simulink library "asbhl20screen"  (R2016b)
settings: Solver=ode45  StartTime=0.0  StopTime=10.0  RelTol=1e-3
undefined symbols (not defined in the file): Tf, Tfg
Description:
  | HL-20 control surface and hydraulic system monitoring modules
settings Model: ExtModeAutoUpdateStatusClock=off  Creator=The MathWorks, Inc.  LastModifiedBy=The MathWorks, Inc.
settings DataIOCC: LimitDataPoints=on  SaveFormat=Array  SignalLoggingSaveFormat=ModelDataLogs
settings OptimizationCC: BlockReduction=off  BooleanDataType=off  ExpressionDepthLimit=2147483647  LifeSpan=inf
settings DebuggingCC: SaveWithParameterizedLinksMsg=none  UnderspecifiedInitializationDetection=Classic  MergeDetectMultiDrivingBlocksExec=none  SignalResolutionControl=TryResolveAllWithWarning  FcnCallInpInsideContextMsg=warning  StateNameClashWarn=warning  StrictBusMsg=Warning  SFUnexpectedBacktrackingDiag=warning  SFNoUnconditionalDefaultTransitionDiag=warning  SFExecutionAtInitializationDiag=none
settings HardwareCC: ProdBitPerPointer=32  ProdBitPerSizeT=32  ProdBitPerPtrDiffT=32  ProdLargestAtomicFloat=None  ProdIntDivRoundTo=Undefined  ProdEndianess=Unspecified  ProdWordSize=32  ProdHWDeviceType=32-bit Generic  TargetUnknown=on
settings ModelReferenceCC: PropagateSignalLabelsOutOfModel=off
settings GRTTargetCC: TargetLangStandard=C89/C90 (ANSI)  GeneratePreprocessorConditionals=Disable all  CombineOutputUpdateFcns=off  GRTInterface=on
settings ConfigComp: CovMetricSettings=dw  CovHtmlReporting=on  CovSaveCumulativeToWorkspaceVar=on  CovSaveSingleToWorkspaceVar=on  CovExternalEMLEnable=off  CovSFcnEnable=off

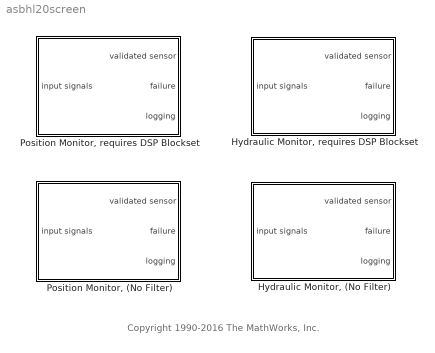
== system asbhl20screen ==
  note: Copyright 1990-2016 The MathWorks, Inc.
  "Hydraulic Monitor, (No Filter)" : Subsystem
  "Hydraulic Monitor, requires DSP Blockset" : Subsystem
  "Position Monitor, (No Filter)" : Subsystem
  "Position Monitor, requires DSP Blockset" : Subsystem

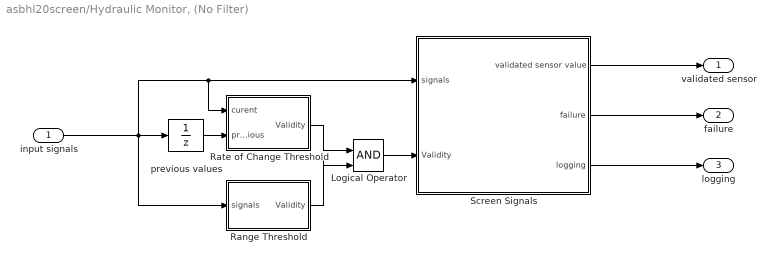
== system asbhl20screen/Hydraulic Monitor, (No Filter) ==
  input signals : Inport  PortDimensions=3  SampleTime=Tf
  Logical Operator : Logic  IconShape=distinctive  AllPortsSameDT=off
  Range Threshold : Subsystem
  Rate of Change Threshold : Subsystem
  Screen Signals : Subsystem
  previous values : UnitDelay  SampleTime=-1
  validated sensor : Outport
  failure : Outport  Port=2
  logging : Outport  Port=3
  wires:
  Screen Signals/3(logging) -> logging/1
  Logical Operator/1 -> Screen Signals/2(Validity)
  Rate of Change Threshold/1(Validity) -> Logical Operator/1
  Range Threshold/1(Validity) -> Logical Operator/2
  previous values/1 -> Rate of Change Threshold/2(previous)
  Screen Signals/1(validated sensor value) -> validated sensor/1
  input signals/1 -> Range Threshold/1(signals), Screen Signals/1(signals), Rate of Change Threshold/1(curent), previous values/1
  Screen Signals/2(failure) -> failure/1

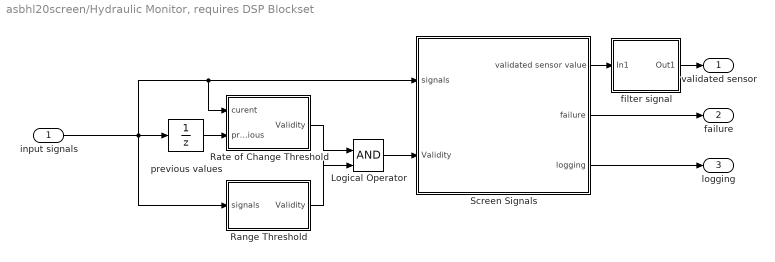
== system asbhl20screen/Hydraulic Monitor, requires DSP Blockset ==
  input signals : Inport  PortDimensions=3  SampleTime=Tf
  Logical Operator : Logic  IconShape=distinctive  AllPortsSameDT=off
  Range Threshold : Subsystem
  Rate of Change Threshold : Subsystem
  Screen Signals : Subsystem
  filter signal : Subsystem
  previous values : UnitDelay  SampleTime=-1
  validated sensor : Outport
  failure : Outport  Port=2
  logging : Outport  Port=3
  wires:
  Screen Signals/2(failure) -> failure/1
  input signals/1 -> previous values/1, Rate of Change Threshold/1(curent), Screen Signals/1(signals), Range Threshold/1(signals)
  Screen Signals/1(validated sensor value) -> filter signal/1(In1)
  previous values/1 -> Rate of Change Threshold/2(previous)
  Range Threshold/1(Validity) -> Logical Operator/2
  Rate of Change Threshold/1(Validity) -> Logical Operator/1
  Logical Operator/1 -> Screen Signals/2(Validity)
  filter signal/1(Out1) -> validated sensor/1
  Screen Signals/3(logging) -> logging/1

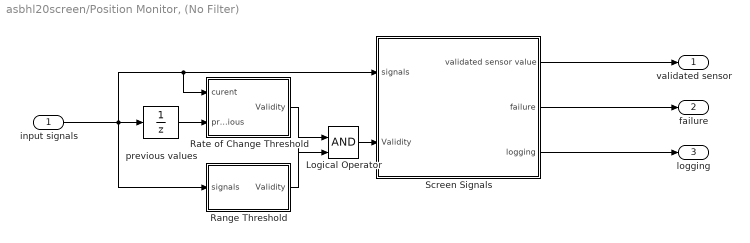
== system asbhl20screen/Position Monitor, (No Filter) ==
  input signals : Inport  PortDimensions=3  SampleTime=Tf
  Logical Operator : Logic  IconShape=distinctive  AllPortsSameDT=off
  Range Threshold : Subsystem
  Rate of Change Threshold : Subsystem
  Screen Signals : Subsystem
  previous values : UnitDelay  SampleTime=-1
  validated sensor : Outport
  failure : Outport  Port=2
  logging : Outport  Port=3
  wires:
  Screen Signals/3(logging) -> logging/1
  Screen Signals/2(failure) -> failure/1
  input signals/1 -> Range Threshold/1(signals), previous values/1, Screen Signals/1(signals), Rate of Change Threshold/1(curent)
  Screen Signals/1(validated sensor value) -> validated sensor/1
  previous values/1 -> Rate of Change Threshold/2(previous)
  Range Threshold/1(Validity) -> Logical Operator/2
  Rate of Change Threshold/1(Validity) -> Logical Operator/1
  Logical Operator/1 -> Screen Signals/2(Validity)

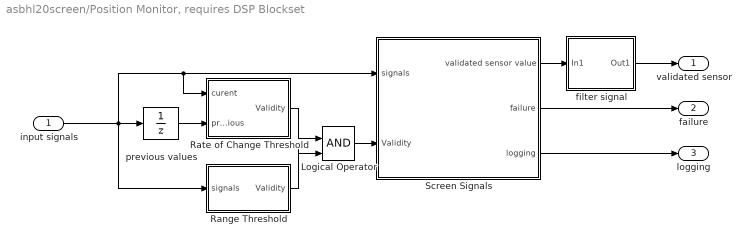
== system asbhl20screen/Position Monitor, requires DSP Blockset ==
  input signals : Inport  PortDimensions=3  SampleTime=Tf
  Logical Operator : Logic  IconShape=distinctive  AllPortsSameDT=off
  Range Threshold : Subsystem
  Rate of Change Threshold : Subsystem
  Screen Signals : Subsystem
  filter signal : Subsystem
  previous values : UnitDelay  SampleTime=-1
  validated sensor : Outport
  failure : Outport  Port=2
  logging : Outport  Port=3
  wires:
  Logical Operator/1 -> Screen Signals/2(Validity)
  Rate of Change Threshold/1(Validity) -> Logical Operator/1
  Range Threshold/1(Validity) -> Logical Operator/2
  previous values/1 -> Rate of Change Threshold/2(previous)
  Screen Signals/1(validated sensor value) -> filter signal/1(In1)
  input signals/1 -> Rate of Change Threshold/1(curent), Screen Signals/1(signals), previous values/1, Range Threshold/1(signals)
  Screen Signals/2(failure) -> failure/1
  Screen Signals/3(logging) -> logging/1
  filter signal/1(Out1) -> validated sensor/1

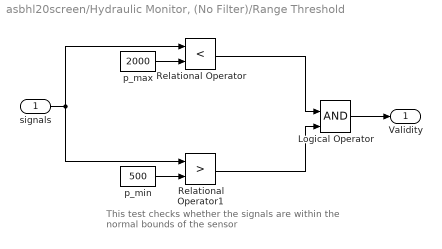
== system asbhl20screen/Hydraulic Monitor, (No Filter)/Range Threshold ==
  note: This test checks whether the signals are within
      | the normal bounds of the sensor
  signals : Inport
  Logical Operator : Logic  IconShape=distinctive  AllPortsSameDT=off
  Relational Operator : RelationalOperator  Operator=<  RndMeth=Nearest
  Relational Operator1 : RelationalOperator  Operator=>  RndMeth=Nearest
  p_max : Constant  Value=2000
  p_min : Constant  Value=500
  Validity : Outport
  wires:
  Logical Operator/1 -> Validity/1
  p_min/1 -> Relational Operator1/2
  p_max/1 -> Relational Operator/2
  Relational Operator1/1 -> Logical Operator/2
  Relational Operator/1 -> Logical Operator/1
  signals/1 -> Relational Operator1/1, Relational Operator/1

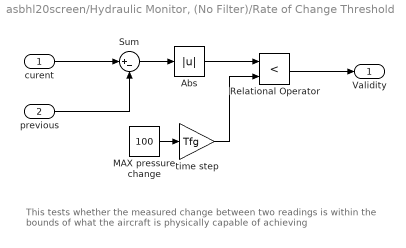
== system asbhl20screen/Hydraulic Monitor, (No Filter)/Rate of Change Threshold ==
  note: This tests whether the measured change between two readings
      | is within the bounds of what the aircraft is physically capable of achieving
  curent : Inport
  previous : Inport  Port=2
  Abs : Abs  SaturateOnIntegerOverflow=on
  MAX pressure change : Constant  Value=100
  Relational Operator : RelationalOperator  Operator=<  OutDataTypeStr=boolean  RndMeth=Nearest
  Sum : Sum  Inputs=|+-  SaturateOnIntegerOverflow=on
  time step : Gain  Gain=Tfg  SaturateOnIntegerOverflow=on  OutDataTypeStr=Inherit: Same as input  ParamDataTypeStr=Inherit: Same as input
  Validity : Outport
  wires:
  Sum/1 -> Abs/1
  time step/1 -> Relational Operator/2
  MAX pressure change/1 -> time step/1
  Relational Operator/1 -> Validity/1
  previous/1 -> Sum/2
  curent/1 -> Sum/1
  Abs/1 -> Relational Operator/1

== system asbhl20screen/Hydraulic Monitor, (No Filter)/Screen Signals ==
  signals : Inport
  Validity : Inport  Port=2
  screen logic : Stateflow chart  TreatAsAtomicUnit=on
  validated sensor value : Outport
  failure : Outport  Port=2
  logging : Outport  Port=3
  wires:
  screen logic/3(" logging") -> logging/1
  signals/1 -> screen logic/1(signals)
  Validity/1 -> screen logic/2(validity)
  screen logic/1(valid_signal) -> validated sensor value/1
  screen logic/2(failure) -> failure/1

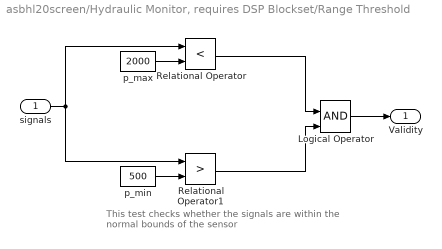
== system asbhl20screen/Hydraulic Monitor, requires DSP Blockset/Range Threshold ==
  note: This test checks whether the signals are within
      | the normal bounds of the sensor
  signals : Inport
  Logical Operator : Logic  IconShape=distinctive  AllPortsSameDT=off
  Relational Operator : RelationalOperator  Operator=<  RndMeth=Nearest
  Relational Operator1 : RelationalOperator  Operator=>  RndMeth=Nearest
  p_max : Constant  Value=2000
  p_min : Constant  Value=500
  Validity : Outport
  wires:
  signals/1 -> Relational Operator/1, Relational Operator1/1
  Relational Operator/1 -> Logical Operator/1
  Relational Operator1/1 -> Logical Operator/2
  p_max/1 -> Relational Operator/2
  p_min/1 -> Relational Operator1/2
  Logical Operator/1 -> Validity/1

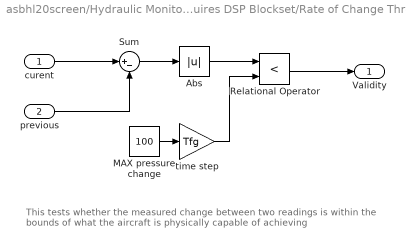
== system asbhl20screen/Hydraulic Monitor, requires DSP Blockset/Rate of Change Threshold ==
  note: This tests whether the measured change between two readings
      | is within the bounds of what the aircraft is physically capable of achieving
  curent : Inport
  previous : Inport  Port=2
  Abs : Abs  SaturateOnIntegerOverflow=on
  MAX pressure change : Constant  Value=100
  Relational Operator : RelationalOperator  Operator=<  OutDataTypeStr=boolean  RndMeth=Nearest
  Sum : Sum  Inputs=|+-  SaturateOnIntegerOverflow=on
  time step : Gain  Gain=Tfg  SaturateOnIntegerOverflow=on  OutDataTypeStr=Inherit: Same as input  ParamDataTypeStr=Inherit: Same as input
  Validity : Outport
  wires:
  curent/1 -> Sum/1
  previous/1 -> Sum/2
  Relational Operator/1 -> Validity/1
  MAX pressure change/1 -> time step/1
  time step/1 -> Relational Operator/2
  Sum/1 -> Abs/1
  Abs/1 -> Relational Operator/1

== system asbhl20screen/Hydraulic Monitor, requires DSP Blockset/Screen Signals ==
  signals : Inport
  Validity : Inport  Port=2
  screen logic : Stateflow chart  TreatAsAtomicUnit=on
  validated sensor value : Outport
  failure : Outport  Port=2
  logging : Outport  Port=3
  wires:
  screen logic/2(failure) -> failure/1
  screen logic/1(valid_signal) -> validated sensor value/1
  Validity/1 -> screen logic/2(validity)
  signals/1 -> screen logic/1(signals)
  screen logic/3(" logging") -> logging/1

== system asbhl20screen/Hydraulic Monitor, requires DSP Blockset/filter signal ==
  In1 : Inport
  Discrete FIR Filter : DiscreteFir  Coefficients=[0.1832 0.3168 0.3168 0.1832]  AccumDataTypeStr=Inherit: Same as product output  OutDataTypeStr=Inherit: Same as input
  Out1 : Outport
  wires:
  In1/1 -> Discrete FIR Filter/1
  Discrete FIR Filter/1 -> Out1/1

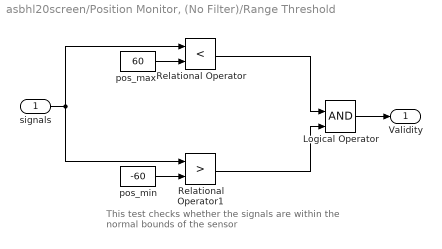
== system asbhl20screen/Position Monitor, (No Filter)/Range Threshold ==
  note: This test checks whether the signals are within
      | the normal bounds of the sensor
  signals : Inport
  Logical Operator : Logic  IconShape=distinctive  AllPortsSameDT=off
  Relational Operator : RelationalOperator  Operator=<  RndMeth=Nearest
  Relational Operator1 : RelationalOperator  Operator=>  RndMeth=Nearest
  pos_max : Constant  Value=60
  pos_min : Constant  Value=-60
  Validity : Outport
  wires:
  Logical Operator/1 -> Validity/1
  pos_min/1 -> Relational Operator1/2
  pos_max/1 -> Relational Operator/2
  Relational Operator1/1 -> Logical Operator/2
  Relational Operator/1 -> Logical Operator/1
  signals/1 -> Relational Operator1/1, Relational Operator/1

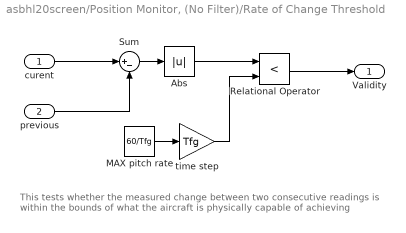
== system asbhl20screen/Position Monitor, (No Filter)/Rate of Change Threshold ==
  note: This tests whether the measured change between two consecutive readings
      | is within the bounds of what the aircraft is physically capable of achieving
  curent : Inport
  previous : Inport  Port=2
  Abs : Abs  SaturateOnIntegerOverflow=on
  MAX pitch rate : Constant  Value=60/Tfg
  Relational Operator : RelationalOperator  Operator=<  OutDataTypeStr=boolean  RndMeth=Nearest
  Sum : Sum  Inputs=|+-  SaturateOnIntegerOverflow=on
  time step : Gain  Gain=Tfg  SaturateOnIntegerOverflow=on  OutDataTypeStr=Inherit: Same as input  ParamDataTypeStr=Inherit: Same as input
  Validity : Outport
  wires:
  curent/1 -> Sum/1
  previous/1 -> Sum/2
  Relational Operator/1 -> Validity/1
  MAX pitch rate/1 -> time step/1
  time step/1 -> Relational Operator/2
  Sum/1 -> Abs/1
  Abs/1 -> Relational Operator/1

== system asbhl20screen/Position Monitor, (No Filter)/Screen Signals ==
  signals : Inport
  Validity : Inport  Port=2
  screen logic : Stateflow chart  TreatAsAtomicUnit=on
  validated sensor value : Outport
  failure : Outport  Port=2
  logging : Outport  Port=3
  wires:
  screen logic/3(" logging") -> logging/1
  screen logic/2(failure) -> failure/1
  screen logic/1(valid_signal) -> validated sensor value/1
  Validity/1 -> screen logic/2(validity)
  signals/1 -> screen logic/1(signals)

== system asbhl20screen/Position Monitor, requires DSP Blockset/Range Threshold ==
  note: This test checks whether the signals are within
      | the normal bounds of the sensor
  signals : Inport
  Logical Operator : Logic  IconShape=distinctive  AllPortsSameDT=off
  Relational Operator : RelationalOperator  Operator=<  RndMeth=Nearest
  Relational Operator1 : RelationalOperator  Operator=>  RndMeth=Nearest
  pos_max : Constant  Value=60
  pos_min : Constant  Value=-60
  Validity : Outport
  wires:
  signals/1 -> Relational Operator/1, Relational Operator1/1
  Relational Operator/1 -> Logical Operator/1
  Relational Operator1/1 -> Logical Operator/2
  pos_max/1 -> Relational Operator/2
  pos_min/1 -> Relational Operator1/2
  Logical Operator/1 -> Validity/1

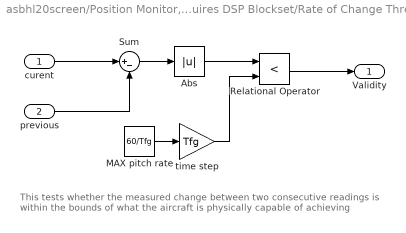
== system asbhl20screen/Position Monitor, requires DSP Blockset/Rate of Change Threshold ==
  note: This tests whether the measured change between two consecutive readings
      | is within the bounds of what the aircraft is physically capable of achieving
  curent : Inport
  previous : Inport  Port=2
  Abs : Abs  SaturateOnIntegerOverflow=on
  MAX pitch rate : Constant  Value=60/Tfg
  Relational Operator : RelationalOperator  Operator=<  OutDataTypeStr=boolean  RndMeth=Nearest
  Sum : Sum  Inputs=|+-  SaturateOnIntegerOverflow=on
  time step : Gain  Gain=Tfg  SaturateOnIntegerOverflow=on  OutDataTypeStr=Inherit: Same as input  ParamDataTypeStr=Inherit: Same as input
  Validity : Outport
  wires:
  Sum/1 -> Abs/1
  time step/1 -> Relational Operator/2
  MAX pitch rate/1 -> time step/1
  Relational Operator/1 -> Validity/1
  previous/1 -> Sum/2
  curent/1 -> Sum/1
  Abs/1 -> Relational Operator/1

== system asbhl20screen/Position Monitor, requires DSP Blockset/Screen Signals ==
  signals : Inport
  Validity : Inport  Port=2
  screen logic : Stateflow chart  TreatAsAtomicUnit=on
  validated sensor value : Outport
  failure : Outport  Port=2
  logging : Outport  Port=3
  wires:
  signals/1 -> screen logic/1(signals)
  Validity/1 -> screen logic/2(validity)
  screen logic/1(valid_signal) -> validated sensor value/1
  screen logic/2(failure) -> failure/1
  screen logic/3(" logging") -> logging/1

== system asbhl20screen/Position Monitor, requires DSP Blockset/filter signal ==
  In1 : Inport
  Discrete FIR Filter : DiscreteFir  Coefficients=[0.1832 0.3168 0.3168 0.1832]  AccumDataTypeStr=Inherit: Same as product output  OutDataTypeStr=Inherit: Same as input
  Out1 : Outport
  wires:
  In1/1 -> Discrete FIR Filter/1
  Discrete FIR Filter/1 -> Out1/1

== stateflow chart asbhl20screen/Position Monitor, (No Filter)/Screen Signals/screen logic ==
  state Screen [parallel]
    settings: executionOrder=1
    note: no valid signals
    state three
      (default) -> (junction 86) : {sum=signals[1]+signals[2]+signals[3];}
      (junction 86) -> (junction 103) : {middle=sum-...
          | max(max(signals[1],signals[2]),signals[3])-...
          | min(min(signals[1],signals[2]),signals[3]);}
      (junction 103) -> (junction 109) [order 1] : [bad==1]
      (junction 109) -> (junction 100) : {none();}
      (junction 103) -> (junction 85) [order 2] : {valid_signal=middle;}
      (junction 85) -> (junction 87) : {failure=0;}
      (junction 87) -> (junction 88) : {prev_signal=valid_signal;}
      (junction 88) -> (junction 108) : {count=0;}
    state zero
      (default) -> (junction 99) : {none();}
    state one
      note: Only one valid sensor - just use the valid signal.
          | Failure is false
      (default) -> (junction 111) : {valid_signal=signals[select[1]];}
      (junction 111) -> (junction 112) : {failure=0;}
      (junction 112) -> (junction 113) : {prev_signal=valid_signal;}
      (junction 113) -> (junction 110) : {count=0;}
    state two
      (default) -> (junction 102) : {diff=abs(signals[select[1]]-signals[select[2]]);}
      (junction 102) -> (junction 107) [order 1] : [diff>diff_max]
      (junction 102) -> (junction 98) [order 2] : {mean=(signals[select[1]]+signals[select[2]])/2;}
      (junction 107) -> (junction 101) : {none();}
      (junction 98) -> (junction 97) : {valid_signal=mean;}
      (junction 97) -> (junction 95) : {failure=0;}
      (junction 95) -> (junction 94) : {prev_signal=valid_signal;}
      (junction 94) -> (junction 106) : {count=0;}
    (default) -> (junction 84) : {n=valid_sensors();}
    three -> Screen
    (junction 84) -> zero [order 4]
    (junction 84) -> three [order 1] : [n==3]
    zero -> Screen
    (junction 84) -> two [order 2] : [n==2]
    (junction 84) -> one [order 3] : [n==1]
    one -> Screen
    two -> Screen
  state failure_logging [parallel]
    settings: executionOrder=2
    state off
    state logging
    off -> logging : log
    logging -> logging [order 2] : log
    (default) -> off
    logging -> off [order 1] : after(30,tick)[~failure]
  state num = valid_sensors() [function]
    (default) -> (junction 228)
    (junction 228) -> (junction 230) : { aVarTruthTableCondition_1 = (validity[1] == 1); }
    (junction 230) -> (junction 232) : { aVarTruthTableCondition_2 = (validity[2] == 1); }
    (junction 232) -> (junction 234) : { aVarTruthTableCondition_3 = (validity[3] == 1); }
    (junction 234) -> (junction 236) [order 1] : [aVarTruthTableCondition_1 && aVarTruthTableCondition_2 && aVarTruthTableCondition_3]
    (junction 236) -> (junction 238) : {
        | /* All 3 signals valid */
        | num = 3;
        | }
    (junction 234) -> (junction 240) [order 2]
    (junction 240) -> (junction 242) [order 1] : [aVarTruthTableCondition_1 && aVarTruthTableCondition_2 && !aVarTruthTableCondition_3]
    (junction 242) -> (junction 244) : {
        | /* Signals 1&2 valid */
        | num = 2;
        | select[1]=1;
        | select[2]=2;
        | }
    (junction 240) -> (junction 246) [order 2]
    (junction 246) -> (junction 248) [order 1] : [aVarTruthTableCondition_1 && !aVarTruthTableCondition_2 && aVarTruthTableCondition_3]
    (junction 248) -> (junction 250) : {
        | /* Signals 1&3 valid */
        | num = 2;
        | select[1]=1;
        | select[2]=3;
        | }
    (junction 246) -> (junction 252) [order 2]
    (junction 252) -> (junction 254) [order 1] : [aVarTruthTableCondition_1 && !aVarTruthTableCondition_2 && !aVarTruthTableCondition_3]
    (junction 254) -> (junction 256) : {
        | /* Signal 1 valid */
        | num = 1;
        | select[1]=1;
        | select[2]=0;
        | }
    (junction 252) -> (junction 258) [order 2]
    (junction 258) -> (junction 260) [order 1] : [!aVarTruthTableCondition_1 && aVarTruthTableCondition_2 && aVarTruthTableCondition_3]
    (junction 260) -> (junction 262) : {
        | /* Signals 2&3 valid */
        | num = 2;
        | select[1]=2;
        | select[2]=3;
        | }
    (junction 258) -> (junction 264) [order 2]
    (junction 264) -> (junction 266) [order 1] : [!aVarTruthTableCondition_1 && aVarTruthTableCondition_2 && !aVarTruthTableCondition_3]
    (junction 266) -> (junction 268) : {
        | /* Signal 2 valid */
        | num = 1;
        | select[1]=2;
        | select[2]=0;
        | }
    (junction 264) -> (junction 270) [order 2]
    (junction 270) -> (junction 272) [order 1] : [!aVarTruthTableCondition_1 && !aVarTruthTableCondition_2 && aVarTruthTableCondition_3]
    (junction 272) -> (junction 274) : {
        | /* Signal 3 valid */
        | num = 1;
        | select[1]=3;
        | select[2]=0;
        | }
    (junction 270) -> (junction 276) [order 2]
    (junction 276) -> (junction 278) [order 1] : [!aVarTruthTableCondition_1 && !aVarTruthTableCondition_2 && !aVarTruthTableCondition_3]
    (junction 278) -> (junction 280) : {
        | /* 'None':no signals valid */
        | num = 0;
        | }
    (junction 276) -> (junction 282) [order 2]
  state none() [function]
    (default) -> (junction 93)
    (junction 93) -> (junction 91) : {count=count+1;}
    (junction 91) -> (junction 104) [order 1] : [count>3]
    (junction 104) -> (junction 92) : {count=3;}
    (junction 92) -> (junction 89) : {valid_signal=0;}
    (junction 91) -> (junction 90) [order 2] : {valid_signal=prev_signal;}
    (junction 89) -> (junction 105) : {failure=1;}
    (junction 90) -> (junction 96) : {failure=0;}
    (junction 96) -> (junction 105) : {send(log,failure_logging)}
  data: middle local double; sum local double; diff local double; mean local double; num function_output int8; aVarTruthTableCondition_1 temporary boolean =0; aVarTruthTableCondition_2 temporary boolean =0; aVarTruthTableCondition_3 temporary boolean =0; signals input double size=3; validity input boolean size=3; n local int8; valid_signal output double; failure output boolean; prev_signal local double; count local int8; diff_max constant double =3; bad local boolean; select local int8 size=2; logging output unknown
  events: log local EITHER_EDGE_EVENT

== stateflow chart asbhl20screen/Hydraulic Monitor, (No Filter)/Screen Signals/screen logic ==
  state Screen [parallel]
    settings: executionOrder=1
    note: no valid signals
    state three
      (default) -> (junction 94) : {sum=signals[1]+signals[2]+signals[3];}
      (junction 94) -> (junction 97) : {middle=sum-...
          | max(max(signals[1],signals[2]),signals[3])-...
          | min(min(signals[1],signals[2]),signals[3]);}
      (junction 97) -> (junction 95) [order 1] : [bad==1]
      (junction 95) -> (junction 98) : {none();}
      (junction 97) -> (junction 101) [order 2] : {valid_signal=middle;}
      (junction 101) -> (junction 102) : {failure=0;}
      (junction 102) -> (junction 107) : {prev_signal=valid_signal;}
      (junction 107) -> (junction 110) : {count=0;}
    state zero
      (default) -> (junction 113) : {none();}
    state one
      note: Only one valid sensor - just use the valid signal.
          | Failure is false
      (default) -> (junction 112) : {valid_signal=signals[select[1]];}
      (junction 112) -> (junction 111) : {failure=0;}
      (junction 111) -> (junction 99) : {prev_signal=valid_signal;}
      (junction 99) -> (junction 108) : {count=0;}
    state two
      (default) -> (junction 87) : {diff=abs(signals[select[1]]-signals[select[2]]);}
      (junction 87) -> (junction 88) [order 1] : [diff>diff_max]
      (junction 87) -> (junction 100) [order 2] : {mean=(signals[select[1]]+signals[select[2]])/2;}
      (junction 88) -> (junction 85) : {none();}
      (junction 100) -> (junction 103) : {valid_signal=mean;}
      (junction 103) -> (junction 109) : {failure=0;}
      (junction 109) -> (junction 86) : {prev_signal=valid_signal;}
      (junction 86) -> (junction 84) : {count=0;}
    (default) -> (junction 106) : {n=valid_sensors();}
    three -> Screen
    (junction 106) -> zero [order 4]
    (junction 106) -> three [order 1] : [n==3]
    zero -> Screen
    (junction 106) -> two [order 2] : [n==2]
    (junction 106) -> one [order 3] : [n==1]
    one -> Screen
    two -> Screen
  state failure_logging [parallel]
    settings: executionOrder=2
    state off
    state logging
    off -> logging : log
    logging -> logging [order 2] : log
    (default) -> off
    logging -> off [order 1] : after(30,tick)[~failure]
  state num = valid_sensors() [function]
    (default) -> (junction 228)
    (junction 228) -> (junction 230) : { aVarTruthTableCondition_1 = (validity[1] == 1); }
    (junction 230) -> (junction 232) : { aVarTruthTableCondition_2 = (validity[2] == 1); }
    (junction 232) -> (junction 234) : { aVarTruthTableCondition_3 = (validity[3] == 1); }
    (junction 234) -> (junction 236) [order 1] : [aVarTruthTableCondition_1 && aVarTruthTableCondition_2 && aVarTruthTableCondition_3]
    (junction 236) -> (junction 238) : {
        | /* All 3 signals valid */
        | num = 3;
        | }
    (junction 234) -> (junction 240) [order 2]
    (junction 240) -> (junction 242) [order 1] : [aVarTruthTableCondition_1 && aVarTruthTableCondition_2 && !aVarTruthTableCondition_3]
    (junction 242) -> (junction 244) : {
        | /* Signals 1&2 valid */
        | num = 2;
        | select[1]=1;
        | select[2]=2;
        | }
    (junction 240) -> (junction 246) [order 2]
    (junction 246) -> (junction 248) [order 1] : [aVarTruthTableCondition_1 && !aVarTruthTableCondition_2 && aVarTruthTableCondition_3]
    (junction 248) -> (junction 250) : {
        | /* Signals 1&3 valid */
        | num = 2;
        | select[1]=1;
        | select[2]=3;
        | }
    (junction 246) -> (junction 252) [order 2]
    (junction 252) -> (junction 254) [order 1] : [aVarTruthTableCondition_1 && !aVarTruthTableCondition_2 && !aVarTruthTableCondition_3]
    (junction 254) -> (junction 256) : {
        | /* Signal 1 valid */
        | num = 1;
        | select[1]=1;
        | select[2]=0;
        | }
    (junction 252) -> (junction 258) [order 2]
    (junction 258) -> (junction 260) [order 1] : [!aVarTruthTableCondition_1 && aVarTruthTableCondition_2 && aVarTruthTableCondition_3]
    (junction 260) -> (junction 262) : {
        | /* Signals 2&3 valid */
        | num = 2;
        | select[1]=2;
        | select[2]=3;
        | }
    (junction 258) -> (junction 264) [order 2]
    (junction 264) -> (junction 266) [order 1] : [!aVarTruthTableCondition_1 && aVarTruthTableCondition_2 && !aVarTruthTableCondition_3]
    (junction 266) -> (junction 268) : {
        | /* Signal 2 valid */
        | num = 1;
        | select[1]=2;
        | select[2]=0;
        | }
    (junction 264) -> (junction 270) [order 2]
    (junction 270) -> (junction 272) [order 1] : [!aVarTruthTableCondition_1 && !aVarTruthTableCondition_2 && aVarTruthTableCondition_3]
    (junction 272) -> (junction 274) : {
        | /* Signal 3 valid */
        | num = 1;
        | select[1]=3;
        | select[2]=0;
        | }
    (junction 270) -> (junction 276) [order 2]
    (junction 276) -> (junction 278) [order 1] : [!aVarTruthTableCondition_1 && !aVarTruthTableCondition_2 && !aVarTruthTableCondition_3]
    (junction 278) -> (junction 280) : {
        | /* 'None':no signals valid */
        | num = 0;
        | }
    (junction 276) -> (junction 282) [order 2]
  state none() [function]
    (default) -> (junction 96)
    (junction 96) -> (junction 105) : {count=count+1;}
    (junction 105) -> (junction 90) [order 1] : [count>3]
    (junction 90) -> (junction 89) : {count=3;}
    (junction 89) -> (junction 92) : {valid_signal=0;}
    (junction 92) -> (junction 93) : {failure=1;}
    (junction 105) -> (junction 91) [order 2] : {valid_signal=prev_signal;}
    (junction 91) -> (junction 104) : {failure=0;}
    (junction 104) -> (junction 93) : {send(log,failure_logging)}
  data: middle local double; sum local double; diff local double; mean local double; num function_output int8; aVarTruthTableCondition_1 temporary boolean =0; aVarTruthTableCondition_2 temporary boolean =0; aVarTruthTableCondition_3 temporary boolean =0; signals input double size=3; validity input boolean size=3; n local int8; valid_signal output double; failure output boolean; prev_signal local double; count local int8; diff_max constant double =10; bad local boolean; select local int8 size=2; logging output unknown
  events: log local EITHER_EDGE_EVENT

== stateflow chart asbhl20screen/Position Monitor, requires DSP Blockset/Screen Signals/screen logic ==
  state Screen [parallel]
    settings: executionOrder=1
    note: no valid signals
    state three
      (default) -> (junction 86) : {sum=signals[1]+signals[2]+signals[3];}
      (junction 86) -> (junction 103) : {middle=sum-...
          | max(max(signals[1],signals[2]),signals[3])-...
          | min(min(signals[1],signals[2]),signals[3]);}
      (junction 103) -> (junction 109) [order 1] : [bad==1]
      (junction 109) -> (junction 100) : {none();}
      (junction 103) -> (junction 85) [order 2] : {valid_signal=middle;}
      (junction 85) -> (junction 87) : {failure=0;}
      (junction 87) -> (junction 88) : {prev_signal=valid_signal;}
      (junction 88) -> (junction 108) : {count=0;}
    state zero
      (default) -> (junction 99) : {none();}
    state one
      note: Only one valid sensor - just use the valid signal.
          | Failure is false
      (default) -> (junction 111) : {valid_signal=signals[select[1]];}
      (junction 111) -> (junction 112) : {failure=0;}
      (junction 112) -> (junction 113) : {prev_signal=valid_signal;}
      (junction 113) -> (junction 110) : {count=0;}
    state two
      (default) -> (junction 102) : {diff=abs(signals[select[1]]-signals[select[2]]);}
      (junction 102) -> (junction 107) [order 1] : [diff>diff_max]
      (junction 102) -> (junction 98) [order 2] : {mean=(signals[select[1]]+signals[select[2]])/2;}
      (junction 107) -> (junction 101) : {none();}
      (junction 98) -> (junction 97) : {valid_signal=mean;}
      (junction 97) -> (junction 95) : {failure=0;}
      (junction 95) -> (junction 94) : {prev_signal=valid_signal;}
      (junction 94) -> (junction 106) : {count=0;}
    (default) -> (junction 84) : {n=valid_sensors();}
    three -> Screen
    (junction 84) -> zero [order 4]
    (junction 84) -> three [order 1] : [n==3]
    zero -> Screen
    (junction 84) -> two [order 2] : [n==2]
    (junction 84) -> one [order 3] : [n==1]
    one -> Screen
    two -> Screen
  state failure_logging [parallel]
    settings: executionOrder=2
    state off
    state logging
    off -> logging : log
    logging -> logging [order 2] : log
    (default) -> off
    logging -> off [order 1] : after(30,tick)[~failure]
  state num = valid_sensors() [function]
    (default) -> (junction 228)
    (junction 228) -> (junction 230) : { aVarTruthTableCondition_1 = (validity[1] == 1); }
    (junction 230) -> (junction 232) : { aVarTruthTableCondition_2 = (validity[2] == 1); }
    (junction 232) -> (junction 234) : { aVarTruthTableCondition_3 = (validity[3] == 1); }
    (junction 234) -> (junction 236) [order 1] : [aVarTruthTableCondition_1 && aVarTruthTableCondition_2 && aVarTruthTableCondition_3]
    (junction 236) -> (junction 238) : {
        | /* All 3 signals valid */
        | num = 3;
        | }
    (junction 234) -> (junction 240) [order 2]
    (junction 240) -> (junction 242) [order 1] : [aVarTruthTableCondition_1 && aVarTruthTableCondition_2 && !aVarTruthTableCondition_3]
    (junction 242) -> (junction 244) : {
        | /* Signals 1&2 valid */
        | num = 2;
        | select[1]=1;
        | select[2]=2;
        | }
    (junction 240) -> (junction 246) [order 2]
    (junction 246) -> (junction 248) [order 1] : [aVarTruthTableCondition_1 && !aVarTruthTableCondition_2 && aVarTruthTableCondition_3]
    (junction 248) -> (junction 250) : {
        | /* Signals 1&3 valid */
        | num = 2;
        | select[1]=1;
        | select[2]=3;
        | }
    (junction 246) -> (junction 252) [order 2]
    (junction 252) -> (junction 254) [order 1] : [aVarTruthTableCondition_1 && !aVarTruthTableCondition_2 && !aVarTruthTableCondition_3]
    (junction 254) -> (junction 256) : {
        | /* Signal 1 valid */
        | num = 1;
        | select[1]=1;
        | select[2]=0;
        | }
    (junction 252) -> (junction 258) [order 2]
    (junction 258) -> (junction 260) [order 1] : [!aVarTruthTableCondition_1 && aVarTruthTableCondition_2 && aVarTruthTableCondition_3]
    (junction 260) -> (junction 262) : {
        | /* Signals 2&3 valid */
        | num = 2;
        | select[1]=2;
        | select[2]=3;
        | }
    (junction 258) -> (junction 264) [order 2]
    (junction 264) -> (junction 266) [order 1] : [!aVarTruthTableCondition_1 && aVarTruthTableCondition_2 && !aVarTruthTableCondition_3]
    (junction 266) -> (junction 268) : {
        | /* Signal 2 valid */
        | num = 1;
        | select[1]=2;
        | select[2]=0;
        | }
    (junction 264) -> (junction 270) [order 2]
    (junction 270) -> (junction 272) [order 1] : [!aVarTruthTableCondition_1 && !aVarTruthTableCondition_2 && aVarTruthTableCondition_3]
    (junction 272) -> (junction 274) : {
        | /* Signal 3 valid */
        | num = 1;
        | select[1]=3;
        | select[2]=0;
        | }
    (junction 270) -> (junction 276) [order 2]
    (junction 276) -> (junction 278) [order 1] : [!aVarTruthTableCondition_1 && !aVarTruthTableCondition_2 && !aVarTruthTableCondition_3]
    (junction 278) -> (junction 280) : {
        | /* 'None':no signals valid */
        | num = 0;
        | }
    (junction 276) -> (junction 282) [order 2]
  state none() [function]
    (default) -> (junction 93)
    (junction 93) -> (junction 91) : {count=count+1;}
    (junction 91) -> (junction 104) [order 1] : [count>3]
    (junction 104) -> (junction 92) : {count=3;}
    (junction 92) -> (junction 89) : {valid_signal=0;}
    (junction 89) -> (junction 105) : {failure=1;}
    (junction 91) -> (junction 90) [order 2] : {valid_signal=prev_signal;}
    (junction 90) -> (junction 96) : {failure=0;}
    (junction 96) -> (junction 105) : {send(log,failure_logging)}
  data: middle local double; sum local double; diff local double; mean local double; diff local double; mean local double; num function_output int8; aVarTruthTableCondition_1 temporary boolean =0; aVarTruthTableCondition_2 temporary boolean =0; aVarTruthTableCondition_3 temporary boolean =0; signals input double size=3; validity input boolean size=3; n local int8; valid_signal output double; failure output boolean; prev_signal local double; count local int8; diff_max constant double =3; bad local boolean; select local int8 size=2; logging output unknown
  events: go_none local EITHER_EDGE_EVENT; continue local EITHER_EDGE_EVENT; log local EITHER_EDGE_EVENT

== stateflow chart asbhl20screen/Hydraulic Monitor, requires DSP Blockset/Screen Signals/screen logic ==
  state Screen [parallel]
    settings: executionOrder=1
    note: no valid signals
    state three
      (default) -> (junction 94) : {sum=signals[1]+signals[2]+signals[3];}
      (junction 94) -> (junction 97) : {middle=sum-...
          | max(max(signals[1],signals[2]),signals[3])-...
          | min(min(signals[1],signals[2]),signals[3]);}
      (junction 97) -> (junction 95) [order 1] : [bad==1]
      (junction 95) -> (junction 98) : {none();}
      (junction 97) -> (junction 101) [order 2] : {valid_signal=middle;}
      (junction 101) -> (junction 102) : {failure=0;}
      (junction 102) -> (junction 107) : {prev_signal=valid_signal;}
      (junction 107) -> (junction 110) : {count=0;}
    state zero
      (default) -> (junction 113) : {none();}
    state one
      note: Only one valid sensor - just use the valid signal.
          | Failure is false
      (default) -> (junction 112) : {valid_signal=signals[select[1]];}
      (junction 112) -> (junction 111) : {failure=0;}
      (junction 111) -> (junction 99) : {prev_signal=valid_signal;}
      (junction 99) -> (junction 108) : {count=0;}
    state two
      (default) -> (junction 87) : {diff=abs(signals[select[1]]-signals[select[2]]);}
      (junction 87) -> (junction 88) [order 1] : [diff>diff_max]
      (junction 87) -> (junction 100) [order 2] : {mean=(signals[select[1]]+signals[select[2]])/2;}
      (junction 88) -> (junction 85) : {none();}
      (junction 100) -> (junction 103) : {valid_signal=mean;}
      (junction 103) -> (junction 109) : {failure=0;}
      (junction 109) -> (junction 86) : {prev_signal=valid_signal;}
      (junction 86) -> (junction 84) : {count=0;}
    (default) -> (junction 106) : {n=valid_sensors();}
    three -> Screen
    (junction 106) -> zero [order 4]
    (junction 106) -> three [order 1] : [n==3]
    zero -> Screen
    (junction 106) -> two [order 2] : [n==2]
    (junction 106) -> one [order 3] : [n==1]
    one -> Screen
    two -> Screen
  state failure_logging [parallel]
    settings: executionOrder=2
    state off
    state logging
    off -> logging : log
    logging -> logging [order 2] : log
    (default) -> off
    logging -> off [order 1] : after(30,tick)[~failure]
  state num = valid_sensors() [function]
    (default) -> (junction 228)
    (junction 228) -> (junction 230) : { aVarTruthTableCondition_1 = (validity[1] == 1); }
    (junction 230) -> (junction 232) : { aVarTruthTableCondition_2 = (validity[2] == 1); }
    (junction 232) -> (junction 234) : { aVarTruthTableCondition_3 = (validity[3] == 1); }
    (junction 234) -> (junction 236) [order 1] : [aVarTruthTableCondition_1 && aVarTruthTableCondition_2 && aVarTruthTableCondition_3]
    (junction 236) -> (junction 238) : {
        | /* All 3 signals valid */
        | num = 3;
        | }
    (junction 234) -> (junction 240) [order 2]
    (junction 240) -> (junction 242) [order 1] : [aVarTruthTableCondition_1 && aVarTruthTableCondition_2 && !aVarTruthTableCondition_3]
    (junction 242) -> (junction 244) : {
        | /* Signals 1&2 valid */
        | num = 2;
        | select[1]=1;
        | select[2]=2;
        | }
    (junction 240) -> (junction 246) [order 2]
    (junction 246) -> (junction 248) [order 1] : [aVarTruthTableCondition_1 && !aVarTruthTableCondition_2 && aVarTruthTableCondition_3]
    (junction 248) -> (junction 250) : {
        | /* Signals 1&3 valid */
        | num = 2;
        | select[1]=1;
        | select[2]=3;
        | }
    (junction 246) -> (junction 252) [order 2]
    (junction 252) -> (junction 254) [order 1] : [aVarTruthTableCondition_1 && !aVarTruthTableCondition_2 && !aVarTruthTableCondition_3]
    (junction 254) -> (junction 256) : {
        | /* Signal 1 valid */
        | num = 1;
        | select[1]=1;
        | select[2]=0;
        | }
    (junction 252) -> (junction 258) [order 2]
    (junction 258) -> (junction 260) [order 1] : [!aVarTruthTableCondition_1 && aVarTruthTableCondition_2 && aVarTruthTableCondition_3]
    (junction 260) -> (junction 262) : {
        | /* Signals 2&3 valid */
        | num = 2;
        | select[1]=2;
        | select[2]=3;
        | }
    (junction 258) -> (junction 264) [order 2]
    (junction 264) -> (junction 266) [order 1] : [!aVarTruthTableCondition_1 && aVarTruthTableCondition_2 && !aVarTruthTableCondition_3]
    (junction 266) -> (junction 268) : {
        | /* Signal 2 valid */
        | num = 1;
        | select[1]=2;
        | select[2]=0;
        | }
    (junction 264) -> (junction 270) [order 2]
    (junction 270) -> (junction 272) [order 1] : [!aVarTruthTableCondition_1 && !aVarTruthTableCondition_2 && aVarTruthTableCondition_3]
    (junction 272) -> (junction 274) : {
        | /* Signal 3 valid */
        | num = 1;
        | select[1]=3;
        | select[2]=0;
        | }
    (junction 270) -> (junction 276) [order 2]
    (junction 276) -> (junction 278) [order 1] : [!aVarTruthTableCondition_1 && !aVarTruthTableCondition_2 && !aVarTruthTableCondition_3]
    (junction 278) -> (junction 280) : {
        | /* 'None':no signals valid */
        | num = 0;
        | }
    (junction 276) -> (junction 282) [order 2]
  state none() [function]
    (default) -> (junction 96)
    (junction 96) -> (junction 105) : {count=count+1;}
    (junction 105) -> (junction 90) [order 1] : [count>3]
    (junction 90) -> (junction 89) : {count=3;}
    (junction 89) -> (junction 92) : {valid_signal=0;}
    (junction 92) -> (junction 93) : {failure=1;}
    (junction 105) -> (junction 91) [order 2] : {valid_signal=prev_signal;}
    (junction 91) -> (junction 104) : {failure=0;}
    (junction 104) -> (junction 93) : {send(log,failure_logging)}
  data: middle local double; sum local double; diff local double; mean local double; diff local double; mean local double; num function_output int8; aVarTruthTableCondition_1 temporary boolean =0; aVarTruthTableCondition_2 temporary boolean =0; aVarTruthTableCondition_3 temporary boolean =0; signals input double size=3; validity input boolean size=3; n local int8; valid_signal output double; failure output boolean; prev_signal local double; count local int8; diff_max constant double =10; bad local boolean; select local int8 size=2; logging output unknown
  events: go_none local EITHER_EDGE_EVENT; continue local EITHER_EDGE_EVENT; log local EITHER_EDGE_EVENT
